simulink model "Fullcar_model"  (R2018b)
settings: Solver=FixedStepAuto  StartTime=0.0  StopTime=inf  FixedStep=0.002  RelTol=1e-3
PreLoadFcn:
  | fullcar_data
values from neighbouring files (symbols this model uses):
  Body_Ixx = 438.7    [fullcar_data.m]
  Body_Iyy = 1447.5    [fullcar_data.m]
  Body_Izz = 1671.2    [fullcar_data.m]
  Body_m = 1106.284    [fullcar_data.m]
  C_max = 4000    [fullcar_data.m]
  C_min = 300    [fullcar_data.m]
  N = L/B    [Fcn_General_Road.m]    (also in Road_Generator_Fullcar_final.m = floor(length(z_Rough_LH)/20); autoSaver.m = length(Road_z))
  s = (cnt - 1)*N    [Road_Generator_Fullcar_final.m]
  sat_limit = 1000    [fullcar_data.m]    (also in skyhook.m = 500)
  TW = 1568*0.001    (= 1.568)    [fullcar_data.m]
  WB = 2650*0.001    (= 2.65)    [fullcar_data.m]
  Whl_m_Frt = 101.488/2    (= 50.744)    [fullcar_data.m]
  Whl_m_Rr = 86.718/2    (= 43.359)    [fullcar_data.m]
  Y = zeros(N,4)    [autoSaver.m]
undefined symbols (not defined in the file or in its folder): X, Z
libraries: nesl_utility x47, sm_lib x44
(part 3 of 5)

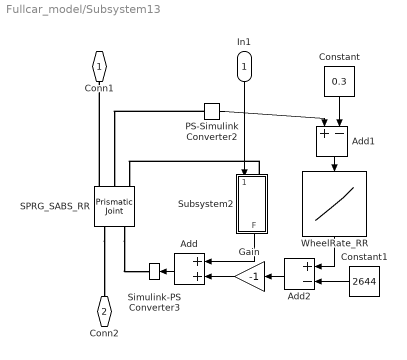
== system Fullcar_model/Subsystem13 ==
  In1 : Inport
  Add : Sum
  Add1 : Sum  Inputs=+-
  Add2 : Sum  Inputs=+-
  Constant : Constant  Value=0.3
  Constant1 : Constant  Value=2644
  Gain : Gain  Gain=-1
  PS-Simulink Converter2 : nesl_utility/PS-Simulink Converter  PhysicalDomain=network_engine_domain  SubClassName=ps_output  LeftPortType=input  RightPortType=output  PseudoPeriodic=off  Frequencies=[]  Unit=1  AffineConversion=off
  SPRG_SABS_RR : sm_lib/Joints/Prismatic Joint  SenseConstraintForce=off  SenseConstraintForceX=off  SenseConstraintForceY=off  SenseConstraintForceZ=off  SenseConstraintTorque=off  SenseConstraintTorqueX=off  SenseConstraintTorqueY=off  SenseConstraintTorqueZ=off  SenseTotalForce=off  SenseTotalForceX=off  SenseTotalForceY=off  SenseTotalForceZ=off  SenseTotalTorque=off  SenseTotalTorqueX=off  SenseTotalTorqueY=off  SenseTotalTorqueZ=off  CompositeWrenchDir=FollowerOnBase  CompositeWrenchFrame=BaseFrame  EquilibriumPosition=0.3  EquilibriumPositionUnits=m  SpringStiffness=0  SpringStiffnessUnits=N/m  DampingCoefficient=0  DampingCoefficientUnits=N/(m/s)  TorqueActuationMode=InputTorque  MotionActuationMode=ComputedMotion  SensePosition=on  SenseVelocity=on  SenseAcceleration=off  SenseTorqueForce=off  PositionTargetSpecify=on  PositionTargetPriority=High  PositionTargetValue=0.3  PositionTargetValueUnits=m  VelocityTargetSpecify=off  VelocityTargetPriority=High  VelocityTargetValue=0  VelocityTargetValueUnits=m/s
  Simulink-PS Converter3 : nesl_utility/Simulink-PS Converter  PhysicalDomain=network_engine_domain  SubClassName=ps_input  LeftPortType=input  RightPortType=output  PseudoPeriodic=off  Frequencies=[]  NoiseDistribution=none  NoiseParameters=[]  Unit=1  AffineConversion=off  FilteringAndDerivatives=provide  SimscapeFilterOrder=1  InputFilterTimeConstant=0.001  UdotUserProvided=0
  Subsystem2 : Subsystem
  WheelRate_RR : Lookup_n-D  NumberOfTableDimensions=1  BreakpointsForDimension1=|  Table=|  InternalRulePriority=Speed  RndMeth=Simplest  InputSameDT=on
      BreakpointsForDimension1=|
      | [-0.0980000000000000
      | -0.0975000000000000
      | -0.0970000000000000
      | -0.0965000000000000
      | -0.0960000000000000
      | -0.0955000000000000
      | -0.0950000000000000
      | -0.0945000000000000
      | -0.0940000000000000
      | -0.0935000000000000
      | -0.0930000000000000
      | -0.0925000000000000
      | -0.0920000000000000
      | -0.0915000000000000
      | -0.0910000000000000
      | -0.0905000000000000
      | -0.0900000000000000
      | -0.0895000000000000
      | -0.0890000000000000
      | -0.0885000000000000
      | -0.0880000000000000
      | -0.0875000000000000
      | -0.0870000000000000
      | -0.0865000000000000
      | -0.0860000000000000
      | -0.0855000000000000
      | -0.0850000000000000
      | -0.0845000000000000
      | -0.0840000000000000
      | -0.0835000000000000
      | -0.0830000000000000
      | -0.0825000000000000
      | -0.0820000000000000
      | -0.0815000000000000
      | -0.0810000000000000
      | -0.0805000000000000
      | -0.0800000000000000
      | -0.0795000000000000
      | -0.0790000000000000
      | -0.0785000000000000
      | -0.0780000000000000
      | -0.0775000000000000
      | -0.0770000000000000
      | -0.0765000000000000
      | -0.0760000000000000
      | -0.0755000000000000
      | -0.0750000000000000
      | -0.0745000000000000
      | -0.0740000000000000
      | -0.0735000000000000
      | -0.0730000000000000
      | -0.0725000000000000
      | -0.0720000000000000
      | -0.0715000000000000
      | -0.0710000000000000
      | -0.0705000000000000
      | -0.0700000000000000
      | -0.0695000000000000
      | -0.0690000000000000
      | -0.0685000000000000
      | -0.0680000000000000
      | -0.0675000000000000
      | -0.0670000000000000
      | -0.0665000000000000
      | -0.0660000000000000
      | -0.0655000000000000
      | -0.0650000000000000
      | -0.0645000000000000
      | -0.0640000000000000
      | -0.0635000000000000
      | -0.0630000000000000
      | -0.0625000000000000
      | -0.0620000000000000
      | -0.0615000000000000
      | -0.0610000000000000
      | -0.0605000000000000
      | -0.0600000000000000
      | -0.0595000000000000
      | -0.0590000000000000
      | -0.0585000000000000
      | -0.0580000000000000
      | -0.0575000000000000
      | -0.0570000000000000
      | -0.0565000000000000
      | -0.0560000000000000
      | -0.0555000000000000
      | -0.0550000000000000
      | -0.0545000000000000
      | -0.0540000000000000
      | -0.0535000000000000
      | -0.0530000000000000
      | -0.0525000000000000
      | -0.0520000000000000
      | -0.0515000000000000
      | -0.0510000000000000
      | -0.0505000000000000
      | -0.0500000000000000
      | -0.0495000000000000
      | -0.0490000000000000
      | -0.0485000000000000
      | -0.0480000000000000
      | -0.0475000000000000
      | -0.0470000000000000
      | -0.0465000000000000
      | -0.0460000000000000
      | -0.0455000000000000
      | -0.0450000000000000
      | -0.0445000000000000
      | -0.0440000000000000
      | -0.0435000000000000
      | -0.0430000000000000
      | -0.0425000000000000
      | -0.0420000000000000
      | -0.0415000000000000
      | -0.0410000000000000
      | -0.0405000000000000
      | -0.0400000000000000
      | -0.0395000000000000
      | -0.0390000000000000
      | -0.0385000000000000
      | -0.0380000000000000
      | -0.0375000000000000
      | -0.0370000000000000
      | -0.0365000000000000
      | -0.0360000000000000
      | -0.0355000000000000
      | -0.0350000000000000
      | -0.0345000000000000
      | -0.0340000000000000
      | -0.0335000000000000
      | -0.0330000000000000
      | -0.0325000000000000
      | -0.0320000000000000
      | -0.0315000000000000
      | -0.0310000000000000
      | -0.0305000000000000
      | -0.0300000000000000
      | -0.0295000000000000
      | -0.0290000000000000
      | -0.0285000000000000
      | -0.0280000000000000
      | -0.0275000000000000
      | -0.0270000000000000
      | -0.0265000000000000
      | -0.0260000000000000
      | -0.0255000000000000
      | -0.0250000000000000
      | -0.0245000000000000
      | -0.0240000000000000
      | -0.0235000000000000
      | -0.0230000000000000
      | -0.0225000000000000
      | -0.0220000000000000
      | -0.0215000000000000
      | -0.0210000000000000
      | -0.0205000000000000
      | -0.0200000000000000
      | -0.0195000000000000
      | -0.0190000000000000
      | -0.0185000000000000
      | -0.0180000000000000
      | -0.0175000000000000
      | -0.0170000000000000
      | -0.0165000000000000
      | -0.0160000000000000
      | -0.0155000000000000
      | -0.0150000000000000
      | -0.0145000000000000
      | -0.0140000000000000
      | -0.0135000000000000
      | -0.0130000000000000
      | -0.0125000000000000
      | -0.0120000000000000
      | -0.0115000000000000
      | -0.0110000000000000
      | -0.0105000000000000
      | -0.0100000000000000
      | -0.00950000000000000
      | -0.00899999999999999
      | -0.00849999999999999
      | -0.00800000000000000
      | -0.00750000000000001
      | -0.00700000000000001
      | -0.00650000000000001
      | -0.00600000000000001
      | -0.00550000000000002
      | -0.00500000000000002
      | -0.00450000000000002
      | -0.00400000000000002
      | -0.00350000000000002
      | -0.00300000000000002
      | -0.00250000000000002
      | -0.00200000000000002
      | -0.00150000000000002
      | -0.00100000000000001
      | -0.000500000000000014
      | -1.38777878078145e-17
      | 0.000499999999999987
      | 0.000999999999999987
      | 0.00149999999999999
      | 0.00199999999999999
      | 0.00249999999999999
      | 0.00299999999999999
      | 0.00349999999999999
      | 0.00399999999999999
      | 0.00449999999999999
      | 0.00499999999999999
      | 0.00549999999999999
      | 0.00599999999999999
      | 0.00649999999999999
      | 0.00699999999999999
      | 0.00749999999999999
      | 0.00799999999999999
      | 0.00849999999999999
      | 0.00899999999999999
      | 0.00950000000000000
      | 0.00999999999999998
      | 0.0105000000000000
      | 0.0110000000000000
      | 0.0115000000000000
      | 0.0120000000000000
      | 0.0125000000000000
      | 0.0130000000000000
      | 0.0135000000000000
      | 0.0140000000000000
      | 0.0145000000000000
      | 0.0150000000000000
      | 0.0155000000000000
      | 0.0160000000000000
      | 0.0165000000000000
      | 0.0170000000000000
      | 0.0175000000000000
      | 0.0180000000000000
      | 0.0185000000000000
      | 0.0190000000000000
      | 0.0195000000000000
      | 0.0200000000000000
      | 0.0205000000000000
      | 0.0210000000000000
      | 0.0215000000000000
      | 0.0220000000000000
      | 0.0225000000000000
      | 0.0230000000000000
      | 0.0235000000000000
      | 0.0240000000000000
      | 0.0245000000000000
      | 0.0250000000000000
      | 0.0255000000000000
      | 0.0260000000000000
      | 0.0265000000000000
      | 0.0270000000000000
      | 0.0275000000000000
      | 0.0280000000000000
      | 0.0285000000000000
      | 0.0290000000000000
      | 0.0295000000000000
      | 0.0300000000000000
      | 0.0305000000000000
      | 0.0310000000000000
      | 0.0315000000000000
      | 0.0320000000000000
      | 0.0325000000000000
      | 0.0330000000000000
      | 0.0335000000000000
      | 0.0340000000000000
      | 0.0345000000000000
      | 0.0350000000000000
      | 0.0355000000000000
      | 0.0360000000000000
      | 0.0365000000000000
      | 0.0370000000000000
      | 0.0375000000000000
      | 0.0380000000000000
      | 0.0385000000000000
      | 0.0390000000000000
      | 0.0395000000000000
      | 0.0400000000000000
      | 0.0405000000000000
      | 0.0410000000000000
      | 0.0415000000000000
      | 0.0420000000000000
      | 0.0425000000000000
      | 0.0430000000000000
      | 0.0435000000000000
      | 0.0440000000000000
      | 0.0445000000000000
      | 0.0450000000000000
      | 0.0455000000000000
      | 0.0460000000000000
      | 0.0465000000000000
      | 0.0470000000000000
      | 0.0475000000000000
      | 0.0480000000000000
      | 0.0485000000000000
      | 0.0490000000000000
      | 0.0495000000000000
      | 0.0500000000000000
      | 0.0505000000000000
      | 0.0510000000000000
      | 0.0515000000000000
      | 0.0520000000000000
      | 0.0525000000000000
      | 0.0530000000000000
      | 0.0535000000000000
      | 0.0540000000000000
      | 0.0545000000000000
      | 0.0550000000000000
      | 0.0555000000000000
      | 0.0560000000000000
      | 0.0565000000000000
      | 0.0570000000000000
      | 0.0575000000000000
      | 0.0580000000000000
      | 0.0585000000000000
      | 0.0590000000000000
      | 0.0595000000000000
      | 0.0600000000000000
      | 0.0605000000000000
      | 0.0610000000000000
      | 0.0615000000000000
      | 0.0620000000000000
      | 0.0625000000000000
      | 0.0630000000000000
      | 0.0635000000000000
      | 0.0640000000000000
      | 0.0645000000000000
      | 0.0650000000000000
      | 0.0655000000000000
      | 0.0660000000000000
      | 0.0665000000000000
      | 0.0670000000000000
      | 0.0675000000000000
      | 0.0680000000000000
      | 0.0685000000000000
      | 0.0690000000000000
      | 0.0695000000000000
      | 0.0700000000000000
      | 0.0705000000000000
      | 0.0710000000000000
      | 0.0715000000000000
      | 0.0720000000000000
      | 0.0725000000000000
      | 0.0730000000000000
      | 0.0735000000000000
      | 0.0740000000000000
      | 0.0745000000000000
      | 0.0750000000000000
      | 0.0755000000000000
      | 0.0760000000000000
      | 0.0765000000000000
      | 0.0770000000000000
      | 0.0775000000000000
      | 0.0780000000000000
      | 0.0785000000000000
      | 0.0790000000000000
      | 0.0795000000000000
      | 0.0800000000000000
      | 0.0805000000000000
      | 0.0810000000000000
      | 0.0815000000000000
      | 0.0820000000000000]
      Table=|
      | [-1435.24406000000
      | -1296.13166000000
      | -1157.01926000000
      | -1017.90686000000
      | -878.794459999998
      | -739.682059999998
      | -600.569659999997
      | -461.457259999997
      | -322.344859999997
      | -183.232459999997
      | -44.1200599999982
      | 22.2150688200019
      | 88.5501976400018
      | 154.885326460002
      | 221.220455280002
      | 287.555584100000
      | 353.890712920000
      | 420.225841740000
      | 486.560970560000
      | 552.896099380000
      | 619.231228200000
      | 630.736880310000
      | 642.242532420000
      | 653.748184530000
      | 665.253836640000
      | 676.759488750000
      | 688.265140860000
      | 699.770792970000
      | 711.276445080000
      | 722.782097190000
      | 734.287749300000
      | 745.793401420000
      | 757.299053540000
      | 768.804705660000
      | 780.310357780000
      | 791.816009900000
      | 803.321662020000
      | 814.827314140000
      | 826.332966260000
      | 837.838618380000
      | 849.344270500000
      | 860.849922610000
      | 872.355574720000
      | 883.861226830000
      | 895.366878940000
      | 906.872531050000
      | 918.378183160000
      | 929.883835270000
      | 941.389487380000
      | 952.895139490001
      | 964.400791600000
      | 975.906443740000
      | 987.412095880001
      | 998.917748020000
      | 1010.42340016000
      | 1021.92905230000
      | 1033.43470444000
      | 1044.94035658000
      | 1056.44600872000
      | 1067.95166086000
      | 1079.45731300000
      | 1090.96296510000
      | 1102.46861720000
      | 1113.97426930000
      | 1125.47992140000
      | 1136.98557350000
      | 1148.49122560000
      | 1159.99687770000
      | 1171.50252980000
      | 1183.00818190000
      | 1194.51383400000
      | 1206.01948610000
      | 1217.52513820000
      | 1229.03079030000
      | 1240.53644240000
      | 1252.04209450000
      | 1263.54774660000
      | 1275.05339870000
      | 1286.55905080000
      | 1298.06470290000
      | 1309.57035500000
      | 1321.07600710000
      | 1332.58165920000
      | 1344.08731130000
      | 1355.59296340000
      | 1367.09861550000
      | 1378.60426760000
      | 1390.10991970000
      | 1401.61557180000
      | 1413.12122390000
      | 1424.62687600000
      | 1436.13252810000
      | 1447.63818020000
      | 1459.14383230000
      | 1470.64948440000
      | 1482.15513650000
      | 1493.66078860000
      | 1505.16644070000
      | 1516.67209280000
      | 1528.17774490000
      | 1539.68339700000
      | 1551.18904910000
      | 1562.69470120000
      | 1574.20035330000
      | 1585.70600540000
      | 1597.21165750000
      | 1608.71730960000
      | 1620.22296170000
      | 1631.72861380000
      | 1643.23426590000
      | 1654.73991800000
      | 1666.24557010000
      | 1677.75122220000
      | 1689.25687430000
      | 1700.76252640000
      | 1712.26817850000
      | 1723.77383060000
      | 1735.27948270000
      | 1746.78513480000
      | 1758.29078690000
      | 1769.79643900000
      | 1781.30209120000
      | 1792.80774340000
      | 1804.31339560000
      | 1815.81904780000
      | 1827.32470000000
      | 1838.83035220000
      | 1850.33600440000
      | 1861.84165660000
      | 1873.34730880000
      | 1884.85296100000
      | 1896.35861310000
      | 1907.86426520000
      | 1919.36991730000
      | 1930.87556940000
      | 1942.38122150000
      | 1953.88687360000
      | 1965.39252570000
      | 1976.89817780000
      | 1988.40382990000
      | 1999.90948200000
      | 2011.41513410000
      | 2022.92078620000
      | 2034.42643830000
      | 2045.93209040000
      | 2057.43774250000
      | 2068.94339460000
      | 2080.44904670000
      | 2091.95469880000
      | 2103.46035090000
      | 2114.96600300000
      | 2126.47165510000
      | 2137.97730720000
      | 2149.48295930000
      | 2160.98861140000
      | 2172.49426350000
      | 2183.99991560000
      | 2195.50556770000
      | 2207.01121980000
      | 2218.51687190000
      | 2230.02252400000
      | 2241.52817610000
      | 2253.03382820000
      | 2264.53948030000
      | 2276.04513240000
      | 2287.55078450000
      | 2299.05643660000
      | 2310.56208870000
      | 2322.06774080000
      | 2333.57339290000
      | 2345.07904500000
      | 2356.58469710000
      | 2368.09034920000
      | 2379.59600130000
      | 2391.10165340000
      | 2402.60730550000
      | 2414.11295760000
      | 2425.61860970000
      | 2437.12426180000
      | 2448.62991390000
      | 2460.13556600000
      | 2471.64121810000
      | 2483.14687020000
      | 2494.65252230000
      | 2506.15817440000
      | 2517.66382650000
      | 2529.16947860000
      | 2540.67513070000
      | 2552.18078280000
      | 2563.68643490000
      | 2575.19208700000
      | 2586.69773910000
      | 2598.20339120000
      | 2609.70904330000
      | 2621.21469540000
      | 2632.72034750000
      | 2644.22599960000
      | 2655.73165170000
      | 2667.23730380000
      | 2678.74295590000
      | 2690.24860800000
      | 2701.75426010000
      | 2713.25991220000
      | 2724.76556430000
      | 2736.27121640000
      | 2747.77686850000
      | 2759.28252060000
      | 2770.78817270000
      | 2782.29382480000
      | 2793.79947690000
      | 2805.30512900000
      | 2816.81078110000
      | 2828.31643320000
      | 2839.82208530000
      | 2851.32773740000
      | 2862.83338950000
      | 2874.33904160000
      | 2885.84469370000
      | 2897.35034580000
      | 2908.85599790000
      | 2920.36165000000
      | 2931.86730210000
      | 2943.37295420000
      | 2954.87860630000
      | 2966.38425840000
      | 2977.88991050000
      | 2989.39556260000
      | 3000.90121470000
      | 3012.40686680000
      | 3023.91251890000
      | 3035.41817100000
      | 3046.92382310000
      | 3058.42947520000
      | 3069.93512730000
      | 3081.44077940000
      | 3092.94643150000
      | 3104.45208360000
      | 3115.95773570000
      | 3127.46338780000
      | 3138.96903990000
      | 3150.47469200000
      | 3161.98034410000
      | 3173.48599620000
      | 3184.99164830000
      | 3196.49730040000
      | 3208.00295250000
      | 3219.50860460000
      | 3231.01425670000
      | 3242.51990880000
      | 3254.02556090000
      | 3265.53121300000
      | 3277.03686510000
      | 3288.54251720000
      | 3300.04816930000
      | 3311.55382140000
      | 3323.05947350000
      | 3334.56512560000
      | 3346.07077770000
      | 3357.57642980000
      | 3369.08208190000
      | 3380.58773400000
      | 3392.09338610000
      | 3403.59903820000
      | 3415.10469030000
      | 3426.61034240000
      | 3438.11599450000
      | 3449.62164660000
      | 3461.12729870000
      | 3472.63295080000
      | 3484.13860290000
      | 3495.64425500000
      | 3512.83848858000
      | 3530.03272216000
      | 3547.22695574000
      | 3564.42118932000
      | 3581.61542290000
      | 3598.80965648000
      | 3616.00389006000
      | 3633.19812364000
      | 3650.39235722000
      | 3667.58659080000
      | 3687.59029079000
      | 3707.59399078000
      | 3727.59769077000
      | 3747.60139076000
      | 3767.60509075000
      | 3787.60879074000
      | 3807.61249073000
      | 3827.61619072000
      | 3847.61989071000
      | 3867.62359070000
      | 3890.77189069000
      | 3913.92019068000
      | 3937.06849067000
      | 3960.21679066000
      | 3983.36509065000
      | 4006.51339064000
      | 4029.66169063000
      | 4052.80999062000
      | 4075.95829061000
      | 4099.10659060000
      | 4125.94489058000
      | 4152.78319056000
      | 4179.62149054000
      | 4206.45979052000
      | 4233.29809050000
      | 4260.13639048000
      | 4286.97469046000
      | 4313.81299044000
      | 4340.65129042000
      | 4367.48959040000
      | 4398.57359039000
      | 4429.65759038000
      | 4460.74159037000
      | 4491.82559036000
      | 4522.90959035000
      | 4553.99359034000
      | 4585.07759033000
      | 4616.16159032000
      | 4647.24559031000
      | 4678.32959030000
      | 4714.21159029000
      | 4750.09359028000
      | 4785.97559026999
      | 4821.85759026000
      | 4857.73959025000
      | 4893.62159024000
      | 4929.50359023000
      | 4965.38559022000
      | 5001.26759021000
      | 5037.14959020000
      | 5097.14959018000
      | 5157.14959016000
      | 5217.14959014000
      | 5277.14959012000
      | 5337.14959010000
      | 5397.14959008000
      | 5457.14959005999
      | 5517.14959004000
      | 5577.14959002000
      | 5637.14959000000
      | 5707.14959000000
      | 5777.14959000000
      | 5847.14959000000
      | 5917.14959000000
      | 5987.14959000000
      | 6057.14959000000
      | 6127.14959000000
      | 6197.14958999999
      | 6267.14959000000
      | 6337.14958999999
      | 6417.14958999999
      | 6497.14959000000
      | 6577.14959000000
      | 6657.14959000000
      | 6737.14959000000
      | 6817.14959000000
      | 6897.14959000000
      | 6977.14959000000
      | 7057.14959000000
      | 7137.14959000000]
  Conn1 : PMIOPort  Side=Right
  Conn2 : PMIOPort  Port=2  Side=Left
  wires:
  In1/1 -> Subsystem2/1("u_RR ")
  Subsystem2/1(F) -> Add/1
  Add/1 -> Simulink-PS Converter3/1
  Add2/1 -> Gain/1
  Constant1/1 -> Add2/2
  WheelRate_RR/1 -> Add2/1
  PS-Simulink Converter2/1 -> Add1/1
  Constant/1 -> Add1/2
  Add1/1 -> WheelRate_RR/1
  Gain/1 -> Add/2
  connections:
  Subsystem2/LConn1 -- SPRG_SABS_RR/RConn3
  SPRG_SABS_RR/LConn2 -- Simulink-PS Converter3/RConn1
  SPRG_SABS_RR/LConn1 -- Conn2/RConn1
  SPRG_SABS_RR/RConn1 -- Conn1/RConn1
  PS-Simulink Converter2/LConn1 -- SPRG_SABS_RR/RConn2
